simulink library "adapt_frame"  (Simulink 5.0)
libraries: dspsigattribs x2, dspbuff3 x2, simulink x2, dspsigops x2, dspmathops x2
settings Model: Creator=dkoh  LastModifiedBy=dkoh

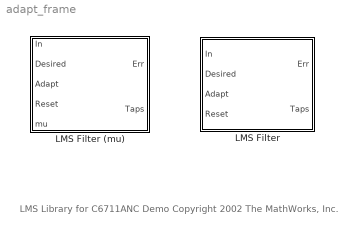
== system adapt_frame ==
  note: LMS Library for C6711ANC Demo
      | Copyright 2002 The MathWorks, Inc.
  LMS Filter : Subsystem  mask(LMS Adaptive Filter){N=32, mu=0.2, leakage=1.0}
      mask prompts: N "Filter Length"; mu "Step Size"
      mask help: Frame-based implementation of a normalized LMS filter.
      mask Display: disp('nLMS\nFrame')
  LMS Filter (mu) : Subsystem  mask(LMS Adaptive Filter){N=32, leakage=1.0}
      mask prompts: N "Filter Length"
      mask help: Frame-based implementation of a normalized LMS filter.
      mask Display: disp('nLMS\nFrame')

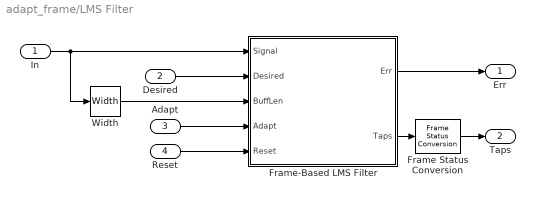
== system adapt_frame/LMS Filter ==
  In : Inport
  Desired : Inport  Port=2
  Adapt : Inport  Port=3
  Reset : Inport  Port=4
  Frame Status Conversion : dspsigattribs/Frame Status Conversion  growRefPort=off  outframe=Sample-based
  Frame-Based LMS Filter : Subsystem  TreatAsAtomicUnit=on
  Width : Width  ShowAdditionalParam=on
  Err : Outport
  Taps : Outport  Port=2
  wires:
  Frame Status Conversion/1 -> Taps/1
  Width/1 -> Frame-Based LMS Filter/3(BuffLen)
  In/1 -> Frame-Based LMS Filter/1(Signal), Width/1
  Desired/1 -> Frame-Based LMS Filter/2(Desired)
  Frame-Based LMS Filter/1(Err) -> Err/1
  Frame-Based LMS Filter/2(Taps) -> Frame Status Conversion/1
  Reset/1 -> Frame-Based LMS Filter/5(Reset)
  Adapt/1 -> Frame-Based LMS Filter/4(Adapt)

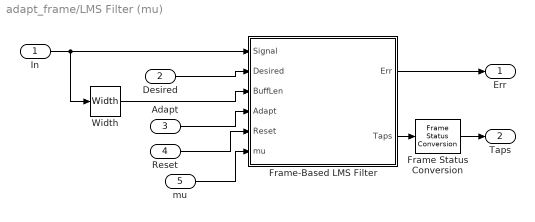
== system adapt_frame/LMS Filter (mu) ==
  In : Inport
  Desired : Inport  Port=2
  Adapt : Inport  Port=3
  Reset : Inport  Port=4
  mu : Inport  Port=5
  Frame Status Conversion : dspsigattribs/Frame Status Conversion  growRefPort=off  outframe=Sample-based
  Frame-Based LMS Filter : Subsystem  TreatAsAtomicUnit=on
  Width : Width  ShowAdditionalParam=on
  Err : Outport
  Taps : Outport  Port=2
  wires:
  Adapt/1 -> Frame-Based LMS Filter/4(Adapt)
  Reset/1 -> Frame-Based LMS Filter/5(Reset)
  Frame-Based LMS Filter/2(Taps) -> Frame Status Conversion/1
  Frame-Based LMS Filter/1(Err) -> Err/1
  Desired/1 -> Frame-Based LMS Filter/2(Desired)
  In/1 -> Width/1, Frame-Based LMS Filter/1(Signal)
  Width/1 -> Frame-Based LMS Filter/3(BuffLen)
  Frame Status Conversion/1 -> Taps/1
  mu/1 -> Frame-Based LMS Filter/6(mu)

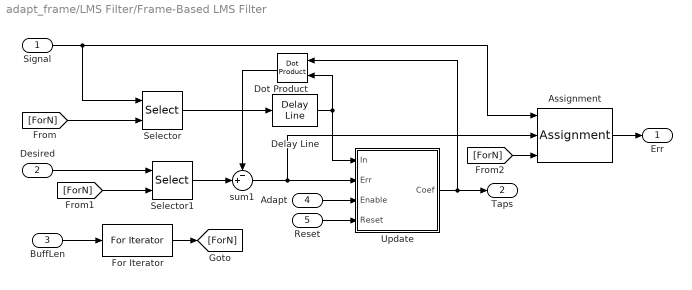
== system adapt_frame/LMS Filter/Frame-Based LMS Filter ==
  Signal : Inport
  Desired : Inport  Port=2
  BuffLen : Inport  Port=3
  Adapt : Inport  Port=4
  Reset : Inport  Port=5
  Assignment : Assignment  ElementSrc=External  Rows=-1  ColumnSrc=External
  Delay Line : dspbuff3/Delay Line  siz=N  ic=0
  Dot Product : simulink/Math Operations/Dot Product  Orientation=left
  For Iterator : ForIterator  IterationSource=external  NumIters=4
  Selector : Selector  ElementSrc=External  Elements=[1 3]
  Selector1 : Selector  ElementSrc=External  Elements=[1 3]
  Update : Subsystem
  sum1 : Sum  Inputs=-+|  SaturateOnIntegerOverflow=on  InputSameDT=on
  Err : Outport
  Taps : Outport  Port=2
  wires:
  Selector1/1 -> sum1/2
  Update/1(Coef) -> Dot Product/1, Taps/1
  Signal/1 -> Selector/1, Assignment/1
  Assignment/1 -> Err/1
  Desired/1 -> Selector1/1
  BuffLen/1 -> For Iterator/1
  Selector/1 -> Delay Line/1
  Delay Line/1 -> Dot Product/2, Update/1(In)
  sum1/1 -> Assignment/2, Update/2(Err)
  Dot Product/1 -> sum1/1
  Adapt/1 -> Update/3(Enable)
  For Iterator/1 -> [ForN]
  [ForN] -> Selector/2
  [ForN] -> Selector1/2
  [ForN] -> Assignment/3
  Reset/1 -> Update/4(Reset)

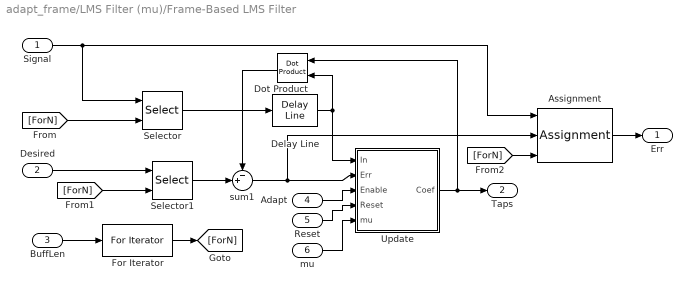
== system adapt_frame/LMS Filter (mu)/Frame-Based LMS Filter ==
  Signal : Inport
  Desired : Inport  Port=2
  BuffLen : Inport  Port=3
  Adapt : Inport  Port=4
  Reset : Inport  Port=5
  mu : Inport  Port=6
  Assignment : Assignment  ElementSrc=External  Rows=-1  ColumnSrc=External
  Delay Line : dspbuff3/Delay Line  siz=N  ic=0
  Dot Product : simulink/Math Operations/Dot Product  Orientation=left
  For Iterator : ForIterator  IterationSource=external  NumIters=4
  Selector : Selector  ElementSrc=External  Elements=[1 3]
  Selector1 : Selector  ElementSrc=External  Elements=[1 3]
  Update : Subsystem
  sum1 : Sum  Inputs=-+|  SaturateOnIntegerOverflow=on  InputSameDT=on
  Err : Outport
  Taps : Outport  Port=2
  wires:
  [ForN] -> Assignment/3
  [ForN] -> Selector1/2
  [ForN] -> Selector/2
  For Iterator/1 -> [ForN]
  Adapt/1 -> Update/3(Enable)
  Dot Product/1 -> sum1/1
  sum1/1 -> Update/2(Err), Assignment/2
  Delay Line/1 -> Update/1(In), Dot Product/2
  Selector/1 -> Delay Line/1
  BuffLen/1 -> For Iterator/1
  Desired/1 -> Selector1/1
  Assignment/1 -> Err/1
  Signal/1 -> Assignment/1, Selector/1
  Update/1(Coef) -> Taps/1, Dot Product/1
  Selector1/1 -> sum1/2
  mu/1 -> Update/5(mu)
  Reset/1 -> Update/4(Reset)

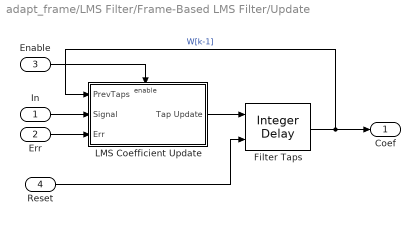
== system adapt_frame/LMS Filter/Frame-Based LMS Filter/Update ==
  In : Inport
  Err : Inport  Port=2
  Enable : Inport  Port=3
  Reset : Inport  Port=4
  Filter Taps : dspsigops/Integer Delay  delay=N  ic=0  reset_popup=Either edge
  LMS Coefficient Update : Subsystem
  Coef : Outport
  wires:
  Err/1 -> LMS Coefficient Update/3(Err)
  Enable/1 -> LMS Coefficient Update/Enable
  In/1 -> LMS Coefficient Update/2(Signal)
  LMS Coefficient Update/1(Tap Update) -> Filter Taps/1
  Filter Taps/1 -> Coef/1, LMS Coefficient Update/1(PrevTaps)  "W[k-1]"
  Reset/1 -> Filter Taps/2

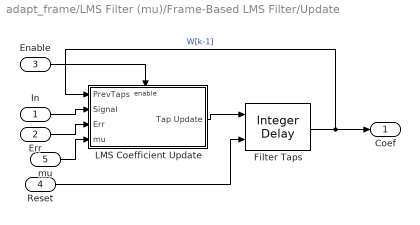
== system adapt_frame/LMS Filter (mu)/Frame-Based LMS Filter/Update ==
  In : Inport
  Err : Inport  Port=2
  Enable : Inport  Port=3
  Reset : Inport  Port=4
  mu : Inport  Port=5
  Filter Taps : dspsigops/Integer Delay  delay=N  ic=0  reset_popup=Either edge
  LMS Coefficient Update : Subsystem
  Coef : Outport
  wires:
  Reset/1 -> Filter Taps/2
  Filter Taps/1 -> LMS Coefficient Update/1(PrevTaps), Coef/1  "W[k-1]"
  LMS Coefficient Update/1(Tap Update) -> Filter Taps/1
  In/1 -> LMS Coefficient Update/2(Signal)
  Enable/1 -> LMS Coefficient Update/Enable
  Err/1 -> LMS Coefficient Update/3(Err)
  mu/1 -> LMS Coefficient Update/4(mu)

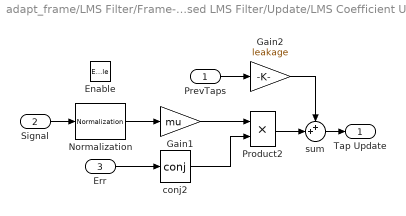
== system adapt_frame/LMS Filter/Frame-Based LMS Filter/Update/LMS Coefficient Update ==
  PrevTaps : Inport
  Signal : Inport  Port=2
  Err : Inport  Port=3
  Enable : EnablePort
  Gain1 : Gain  Gain=mu  SaturateOnIntegerOverflow=on
  Gain2 : Gain  Gain=leakage  SaturateOnIntegerOverflow=on
  Normalization : dspmathops/Normalization  NormType=Squared 2-norm  Bias=1e-10
  Product2 : Product  SaturateOnIntegerOverflow=on  InputSameDT=on
  conj2 : Math  Operator=conj
  sum : Sum  Inputs=++|  SaturateOnIntegerOverflow=on  InputSameDT=on
  Tap Update : Outport  InitialOutput=0
  wires:
  conj2/1 -> Product2/2
  Normalization/1 -> Gain1/1
  Signal/1 -> Normalization/1
  Err/1 -> conj2/1
  Product2/1 -> sum/2
  sum/1 -> Tap Update/1
  PrevTaps/1 -> Gain2/1
  Gain2/1 -> sum/1
  Gain1/1 -> Product2/1

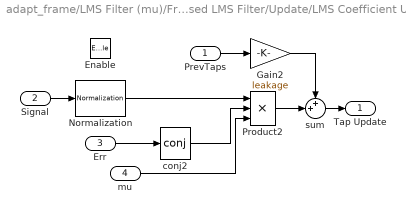
== system adapt_frame/LMS Filter (mu)/Frame-Based LMS Filter/Update/LMS Coefficient Update ==
  PrevTaps : Inport
  Signal : Inport  Port=2
  Err : Inport  Port=3
  mu : Inport  Port=4
  Enable : EnablePort
  Gain2 : Gain  Gain=leakage  SaturateOnIntegerOverflow=on
  Normalization : dspmathops/Normalization  NormType=Squared 2-norm  Bias=1e-10
  Product2 : Product  Inputs=3  SaturateOnIntegerOverflow=on  InputSameDT=on
  conj2 : Math  Operator=conj
  sum : Sum  Inputs=++|  SaturateOnIntegerOverflow=on  InputSameDT=on
  Tap Update : Outport  InitialOutput=0
  wires:
  Gain2/1 -> sum/1
  PrevTaps/1 -> Gain2/1
  sum/1 -> Tap Update/1
  Product2/1 -> sum/2
  Err/1 -> conj2/1
  Signal/1 -> Normalization/1
  Normalization/1 -> Product2/1
  conj2/1 -> Product2/2
  mu/1 -> Product2/3
